simulink model "Host_model_Rotor_pos_est"  (R2021b)
settings: Solver=FixedStepDiscrete  StartTime=0.0  StopTime=Inf  RelTol=1e-3  EnableMultiTasking=on
model workspace (MAT data in the model file):
  estimator = 1
values from neighbouring files (symbols this model uses):
  Ts = 1/(8*fsw)    (= 1.25e-05)    [init.m]
libraries: mcbhostblockslib x3
PreSaveFcn:
  | if( strcmp(get_param([gcs '/TX/HW_Selected'], 'Value'), '0'))
  |       set_param([gcs '/Host Serial Setup'], 'baudRateA', '5.625e6');
  | elseif( strcmp(get_param([gcs '/TX/HW_Selected'], 'Value'), '1'))
  |       set_param([gcs '/Host Serial Setup'], 'baudRateA', '5e6');
  | end
settings Model: ExtModeTrigDuration=8  Creator=The MathWorks, Inc.  LastModifiedBy=jussi
settings SolverCC: AlgebraicLoopSolver=TrustRegion
settings DataIOCC: LimitDataPoints=on  SaveFormat=Array  ReturnWorkspaceOutputs=off
settings OptimizationCC: DefaultUnderspecifiedDataType=single  LifeSpan=1  MaxStackSize=1024  DenormalBehavior=FlushToZero  EfficientTunableParamExpr=on
settings DebuggingCC: UnderspecifiedInitializationDetection=Classic  MergeDetectMultiDrivingBlocksExec=none  SolverPrmCheckMsg=warning  ParameterPrecisionLossMsg=none  AllowSymbolicDim=off  PregeneratedLibrarySubsystemCodeDiagnostic=none  SFUnexpectedBacktrackingDiag=warning  SFNoUnconditionalDefaultTransitionDiag=warning  SFExecutionAtInitializationDiag=none  SFMachineParentedDataDiag=warning  ArithmeticOperatorsInVariantConditions=warning
settings HardwareCC: ProdBitPerChar=16  ProdBitPerInt=16  ProdBitPerPointer=32  ProdBitPerSizeT=32  ProdBitPerPtrDiffT=32  ProdLargestAtomicInteger=Integer  ProdLargestAtomicFloat=None  ProdWordSize=16  ProdLongLongMode=on  ProdHWDeviceType=Texas Instruments->C2000
settings ModelReferenceCC: PropagateSignalLabelsOutOfModel=off
settings SFSimCC: SimUseLocalCustomCode=off  MATLABDynamicMemAlloc=off
settings RTWCC: Description=Real-Time Workshop Embedded Coder  SystemTargetFile=ert.tlc  HardwareBoard=TI Delfino F28379D LaunchPad  TemplateMakefile=ert_default_tmf  GenerateReport=on  RTWUseLocalCustomCode=off  Toolchain=Texas Instruments Code Composer Studio (C2000)  IncludeHyperlinkInReport=on  LaunchReport=on  GenerateTraceInfo=on  GenerateTraceReport=on  GenerateTraceReportSl=on  GenerateTraceReportSf=on  GenerateTraceReportEml=on
settings CodeAppCC: IgnoreCustomStorageClasses=off  StateflowObjectComments=on  InternalIdentifier=Classic
settings ERTTargetCC: CodeReplacementLibrary=TI C28x  MultiwordLength=2048  ExtModeStaticAllocSize=10000  ConvertIfToSwitch=off  SuppressUnreachableDefaultCases=off
settings ConfigComp: CovMetricSettings=dw  CovSaveCumulativeToWorkspaceVar=on  CovSaveSingleToWorkspaceVar=on  CovExternalEMLEnable=off  CovSFcnEnable=off

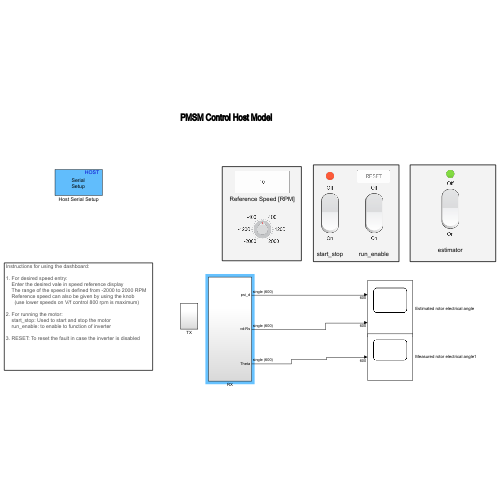
[thumbnail: Simulink's stored preview of the top-level diagram]
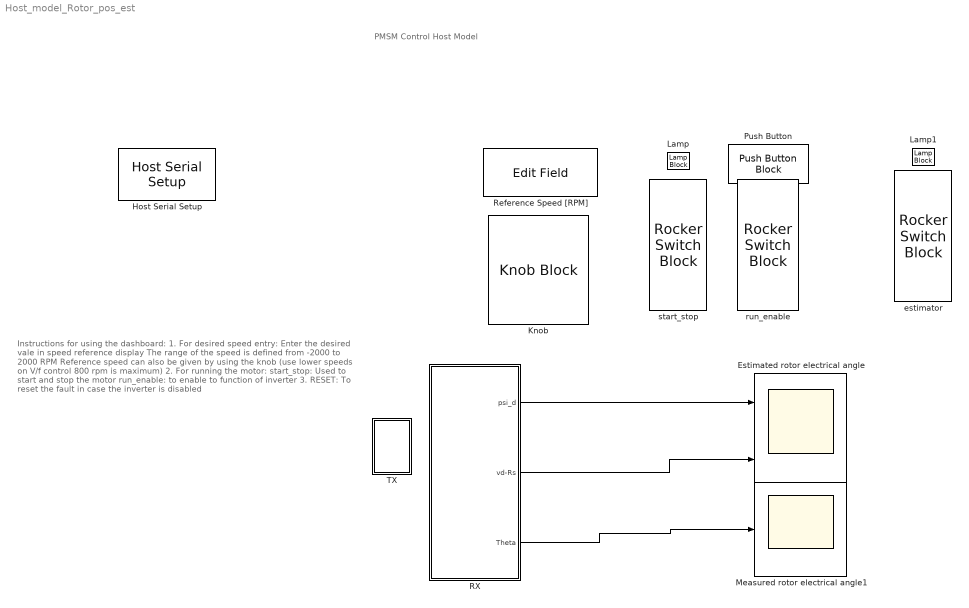
== system Host_model_Rotor_pos_est ==
  note: Instructions for using the dashboard:
      |
      | 1. For desired speed entry:
      |     Enter the desired vale in speed reference display
      |     The range of the speed is defined from -2000 to 2000 RPM
      |     Reference speed can also be given by using the knob
      | 	(use lower speeds on V/f control 800 rpm is maximum)
      |
      | 2. For running the motor:
      |     start_stop: Used to start and stop the motor
      |     run_enable: to enable to function of inverter
      |
      | 3. RESET: To reset the fault in case the inverter is disabled
  note: PMSM Control Host Model
  Estimated rotor electrical angle : Scope  NumInputPorts=2
  Host Serial Setup : mcbhostblockslib/Host Serial Setup  Priority=-99  comPortSer1='COM4'  baudRateA=5e6  charLenA=8  stopBitA=1  parityA=none  timeoutA=2  ByteOrderA=LittleEndian  comPortSer2='Please_select_a_port'  baudRateB=115200  charLenB=8  stopBitB=1  parityB=none  timeoutB=1.0  ByteOrderB=LittleEndian  comPortSer3='Please_select_a_port'  baudRateC=115200  charLenC=8  stopBitC=1  parityC=none  timeoutC=1.0  ByteOrderC=LittleEndian  comPortSer4='Please_select_a_port'  baudRateD=115200  charLenD=8  stopBitD=1  parityD=none  timeoutD=1.0  ByteOrderD=LittleEndian
      settings: SourceProductBaseCode=MT
  Knob : KnobBlock  LabelPosition=Hide  ScaleMin=-2000  ScaleMax=2000
  Lamp : LampBlock  LabelPosition=Hide
  Lamp1 : LampBlock  LabelPosition=Hide
  Measured rotor electrical angle1 : Scope
  Push Button : PushButtonBlock  ButtonText=RESET  OffValue=0.000000
  RX : Subsystem
  Reference Speed [RPM] : EditField  LabelPosition=Hide  ShowInitialText=on  Alignment=Center
  TX : Subsystem
  estimator : RockerSwitchBlock  LabelPosition=Hide
      settings: Values={{'On', 'Off'}, [1 0]}
  run_enable : RockerSwitchBlock  LabelPosition=Hide
      settings: Values={{'On', 'Off'}, [1 0]}
  start_stop : RockerSwitchBlock  LabelPosition=Hide
      settings: Values={{'On', 'Off'}, [1 0]}
  wires:
  RX/3(Theta) -> Measured rotor electrical angle1/1
  RX/1(psi_d) -> Estimated rotor electrical angle/1
  RX/2(vd-Rs) -> Estimated rotor electrical angle/2

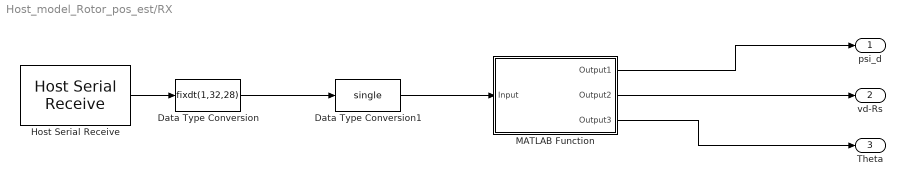
== system Host_model_Rotor_pos_est/RX ==
  Data Type Conversion : DataTypeConversion  OutDataTypeStr=fixdt(1,32,28)  ConvertRealWorld=Stored Integer (SI)  RndMeth=Simplest
  Data Type Conversion1 : DataTypeConversion  OutDataTypeStr=single  RndMeth=Simplest
  Host Serial Receive : mcbhostblockslib/Host Serial Receive  serialCon=Serial 1  dataHead='SSSS'  dataTail='EEEE'  dataType=uint32  dataDim=[600 3]  initValue=5  errOption=Output custom value  errValue=4  sampleTime=600*Ts  outputStatus=off  blockingMode=on
      settings: SourceProductBaseCode=MT
  MATLAB Function : MATLAB Function  TreatAsAtomicUnit=on
  psi_d : Outport
  vd-Rs : Outport  Port=2
  Theta : Outport  Port=3
  wires:
  Data Type Conversion/1 -> Data Type Conversion1/1
  Host Serial Receive/1 -> Data Type Conversion/1
  Data Type Conversion1/1 -> MATLAB Function/1(Input)
  MATLAB Function/1(Output1) -> psi_d/1
  MATLAB Function/3(Output3) -> Theta/1
  MATLAB Function/2(Output2) -> vd-Rs/1

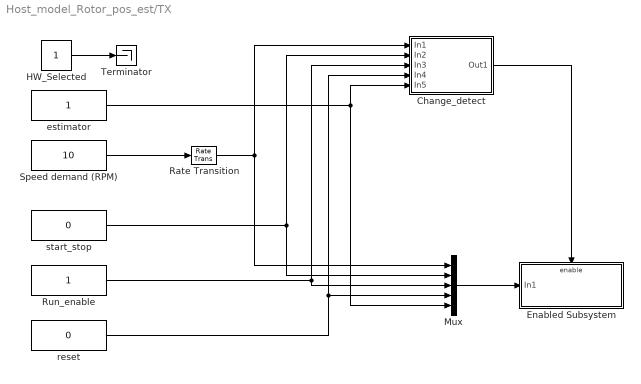
== system Host_model_Rotor_pos_est/TX ==
  Change_detect : Subsystem
  Enabled Subsystem : Subsystem  TreatAsAtomicUnit=on
  HW_Selected : Constant  OutDataTypeStr=uint8
  Mux : Mux  Inputs=5
  Rate Transition : RateTransition  OutPortSampleTime=0.03
  Run_enable : Constant  VectorParams1D=off  OutDataTypeStr=single  SampleTime=0.03
  Speed demand (RPM) : Constant  Value=10  VectorParams1D=off  OutDataTypeStr=single  SampleTime=0.03
  Terminator : Terminator
  estimator : Constant  VectorParams1D=off  OutDataTypeStr=single  SampleTime=0.03
  reset : Constant  Value=0  VectorParams1D=off  OutDataTypeStr=single  SampleTime=0.03
  start_stop : Constant  Value=0  VectorParams1D=off  OutDataTypeStr=single  SampleTime=0.03
  wires:
  start_stop/1 -> Mux/2, Change_detect/2(In2)
  Speed demand (RPM)/1 -> Rate Transition/1
  Mux/1 -> Enabled Subsystem/1(In1)
  Rate Transition/1 -> Mux/1, Change_detect/1(In1)
  Change_detect/1(Out1) -> Enabled Subsystem/Enable
  HW_Selected/1 -> Terminator/1
  Run_enable/1 -> Mux/3, Change_detect/3(In3)
  reset/1 -> Mux/4, Change_detect/4(In4)
  estimator/1 -> Mux/5, Change_detect/5(In5)

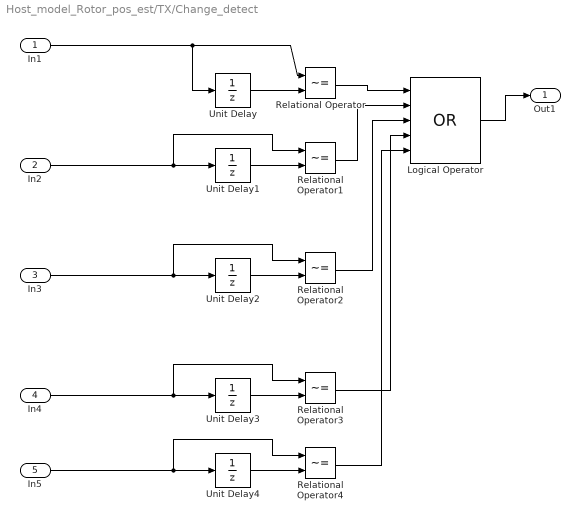
== system Host_model_Rotor_pos_est/TX/Change_detect ==
  In1 : Inport
  In2 : Inport  Port=2
  In3 : Inport  Port=3
  In4 : Inport  Port=4
  In5 : Inport  Port=5
  Logical Operator : Logic  Operator=OR  Inputs=5  AllPortsSameDT=off  OutDataTypeStr=boolean
  Relational Operator{,1..4} (5 alike) : RelationalOperator  Operator=~=  OutDataTypeStr=boolean  RndMeth=Nearest
  Unit Delay : UnitDelay  InitialCondition=0.5  SampleTime=-1  HasFrameUpgradeWarning=on
  Unit Delay{1..4} (4 alike) : UnitDelay  SampleTime=-1  HasFrameUpgradeWarning=on
  Out1 : Outport  VectorParamsAs1DForOutWhenUnconnected=off
  wires:
  In2/1 -> Relational Operator1/1, Unit Delay1/1
  Relational Operator1/1 -> Logical Operator/2
  Unit Delay1/1 -> Relational Operator1/2
  Unit Delay/1 -> Relational Operator/2
  In1/1 -> Unit Delay/1, Relational Operator/1
  Relational Operator/1 -> Logical Operator/1
  Logical Operator/1 -> Out1/1
  In3/1 -> Relational Operator2/1, Unit Delay2/1
  Relational Operator2/1 -> Logical Operator/3
  Unit Delay2/1 -> Relational Operator2/2
  In4/1 -> Relational Operator3/1, Unit Delay3/1
  Relational Operator3/1 -> Logical Operator/4
  Unit Delay3/1 -> Relational Operator3/2
  In5/1 -> Relational Operator4/1, Unit Delay4/1
  Unit Delay4/1 -> Relational Operator4/2
  Relational Operator4/1 -> Logical Operator/5

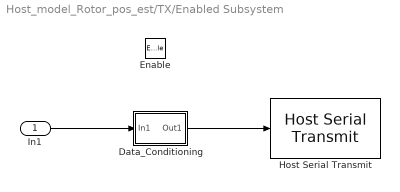
== system Host_model_Rotor_pos_est/TX/Enabled Subsystem ==
  In1 : Inport
  Enable : EnablePort
  Data_Conditioning : Subsystem
  Host Serial Transmit : mcbhostblockslib/Host Serial Transmit  serialCon=Serial 1  header=''  tail=''  enableBlockingMode=off
      settings: SourceProductBaseCode=MT
  wires:
  In1/1 -> Data_Conditioning/1(In1)
  Data_Conditioning/1(Out1) -> Host Serial Transmit/1

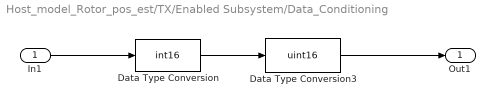
== system Host_model_Rotor_pos_est/TX/Enabled Subsystem/Data_Conditioning ==
  In1 : Inport
  Data Type Conversion : DataTypeConversion  OutDataTypeStr=int16  RndMeth=Simplest
  Data Type Conversion3 : DataTypeConversion  OutDataTypeStr=uint16  ConvertRealWorld=Stored Integer (SI)  RndMeth=Simplest
  Out1 : Outport  VectorParamsAs1DForOutWhenUnconnected=off
  wires:
  In1/1 -> Data Type Conversion/1
  Data Type Conversion3/1 -> Out1/1
  Data Type Conversion/1 -> Data Type Conversion3/1

== matlab function Host_model_Rotor_pos_est/RX/MATLAB Function ==
  data: Output1 output; Output2 output; Input input; Output3 output
function [ Output1, Output2, Output3] = unBuf(Input)

Output1= Input(:, 1);
Output2 = Input(:, 2);
Output3 = Input(:, 3);
end
